simulink model "SIL_Microgrid"  (R2024a)
settings: Solver=FixedStepDiscrete  StartTime=0.0  StopTime=10  FixedStep=T_simulation  RelTol=1e-3
model workspace (MAT data in the model file):
  ICAR = 3200
  ICR = 3200
  P_0 = 0
  P_s = 10000
  Q_0 = 0
  Q_s = 1000
  T_f_VI = 0.1
  T_sampleFFR = 0.01
  T_simulation = 0.001
  batteryCellCapacity_Ah = 2
  m_p_VI = 0.1
  numberCellsParallel = 1
  numberCellsSerial = 200
libraries: spsControlledCurrentSourceLib x6, spsThreePhaseVIMeasurementLib x4, spsControlledVoltageSourceLib x3, spsGroundLib x3, spsThreePhaseParallelRLCBranchLib x3, spsThreePhaseSeriesRLCBranchLib x3, eeGeneralControl x2, simulink_extras x2, spsThreePhaseSineGeneratorLib x2, eeSinGeneratorThreePhase x1, eePowerMeasurement x1, sps_lib x1
(part 2 of 2)

== matlab function SIL_Microgrid/Subsystem_AncillaryServices/Subsystem_FFR_and_VoltageSupport/ROCOF_FFR2_MATLAB_Function ==
  data: freq input; rocof output; time input; threshold input; tr input
% This function computes the rate of change of frequency (RoCoF) over a
% 500ms window only after it has been triggered by the incremental df/dt
% being below or equal to the transfer parameter "threshold". 
% The particular RoCoF will be returned for 30 seconds and return zeros 
% until it is triggered again.
%
%##### Input description #####
% freq     : freqency input (Hz)
% time     : time input (s)
% threshold: for triggering the rocof calculation over 500ms shall be negative and in Hz/s
% tr       : must be the same as the time resolution of the simulation, i.e. step size (typ. 0.1s, max. 0.5s).
%##### Output description #####
% rocof: standard output is zero. After the incremental difference df/dt falls
%        below the threshold value, the algorithm starts calculating the
%        rocof over a 0.5s window and outputs it as soon as available.

function rocof = ROCOF_FFR2(freq, time, threshold, tr) 
%% Definition of persistent variables
persistent fcurrent;
if isempty(fcurrent)
    fcurrent = freq;
end

persistent tcurrent;
if isempty(tcurrent)
    tcurrent = -1;
end

persistent fminus1;
persistent tminus1;

persistent isTriggered;
if isempty(isTriggered)
    isTriggered = false;
end

persistent tTriggered;
if isempty(tTriggered)
    tTriggered=-31;
end

persistent rollingWindow;
if isempty(rollingWindow)
    rollingWindow = zeros(0.5/tr,2); % Creating the rolling window with 2 columns and 0.5s/tr rows, e.g. for tr=0.1s 5 rows
end

%% Start of algorithm
    tminus1 = tcurrent;
    tcurrent = time;
    fminus1 = fcurrent;
    fcurrent = freq;

    if isTriggered == false % Incremental difference one step until triggered
        rocof = 0;

        df = fcurrent-fminus1;
        dt = tcurrent-tminus1;
        dfdt = df/dt;
    
        if dfdt <= threshold
            isTriggered = true;
            tTriggered = tminus1;
            rollingWindow(1,:)=[tminus1,fminus1];
            rollingWindow(2,:)=[tcurrent,fcurrent];
        end
    else % isTriggered == true
        if (tcurrent-tTriggered) >= 29.9999 % cannot use ">= 30" due to limited exactness
            isTriggered = false;
            rocof = 0;
        elseif (tcurrent-tTriggered) >= 0.4999 % cannot use ">= 0.5" due to limited exactness
            fminus500ms = rollingWindow(mod((round((tcurrent-0.5-tTriggered)/tr)),round(0.5/tr))+1,2);
            rocof = (fcurrent - fminus500ms)/0.5; % calculate rocof over a 0.5s = 500ms window
            % store the current time and frequency values
            rollingWindow(mod((round((tcurrent-0.5-tTriggered)/tr)),round(0.5/tr))+1,:) = [tcurrent,fcurrent];
        else % (tcurrent-tTriggered) < 0.5
            rocof = 0; % ride-through for the first 500 ms after trigger event, i.e. before the rolling window is operable
            % store the current time and frequency values
            rollingWindow((round((tcurrent-tTriggered)/tr))+1,:) = [tcurrent,fcurrent];
        end
    end
end

== matlab function SIL_Microgrid/Subsystem_AncillaryServices/Subsystem_FFR_and_VoltageSupport/ROCOF_FFR4_MATLAB_Function ==
  data: freq input; rocof output; time input
% This function computes the rate of change of frequency (RoCoF) in Hz/s 
% of one sample based on the previous sample. 
% 
%##### Input description #####
% freq: freqency input (Hz)
% time: time input (seconds)
%##### Output description #####
% rocof: Output is the derivative of freq, i.e. the quotient of the
% difference between the current and previous step in frequency and time: 
% delta_f/delta_t.

function rocof = ROCOF_FFR4(freq, time) 
%% Definition of persistent variables
persistent fcurrent;
if isempty(fcurrent)
    fcurrent = freq;
end

persistent tcurrent;
if isempty(tcurrent)
    tcurrent = -1;
end

persistent fminus1;
persistent tminus1;
%% Start of algorithm
    tminus1 = tcurrent;
    tcurrent = time;
    fminus1 = fcurrent;
    fcurrent = freq;

    % Incremental difference one step until triggered
    delta_f = fcurrent-fminus1;
    delta_t = tcurrent-tminus1;
    rocof = delta_f/delta_t;
end
